simulink model "simulink_model"  (R2023b)
settings: Solver=VariableStepAuto  StartTime=0.0  StopTime=Inf  RelTol=1e-3
values from neighbouring files (symbols this model uses):
  A = [-1.064 1.000; 290.26 0.00]    [model.m]
  B = [-0.25; -331.40]    [model.m]
  C = [-123.34 0.00; 0.00 1.00]    [model.m]
  D = [-13.51; 0]    [model.m]
  dT1 = 0.75    [model.m]
  dT2 = 0.25    [model.m]
  ELEV_INIT = 10000    [model.m]
  ELEV_TARGET = 795    [model.m]
  LAT_INIT = 34.2329    [model.m]
  LAT_OBS = 34.61916    [model.m]
  LAT_TARGET = 34.6588    [model.m]
  LON_INIT = -119.4573    [model.m]
  LON_OBS = -118.8429    [model.m]
  LON_TARGET = -118.769745    [model.m]
  Vel = 1021.08    [model.m]
undefined symbols (not defined in the file or in its folder): Earth, K, L, WGS84
libraries: simulink x3, aerolibtransform2 x1, slpidlib x1, aerolibanimutils x1
settings Model: Creator=Arseni  LastModifiedBy=Arseni

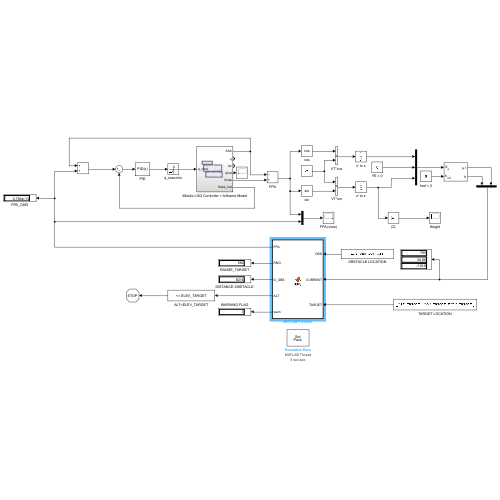
[thumbnail: Simulink's stored preview of the top-level diagram]
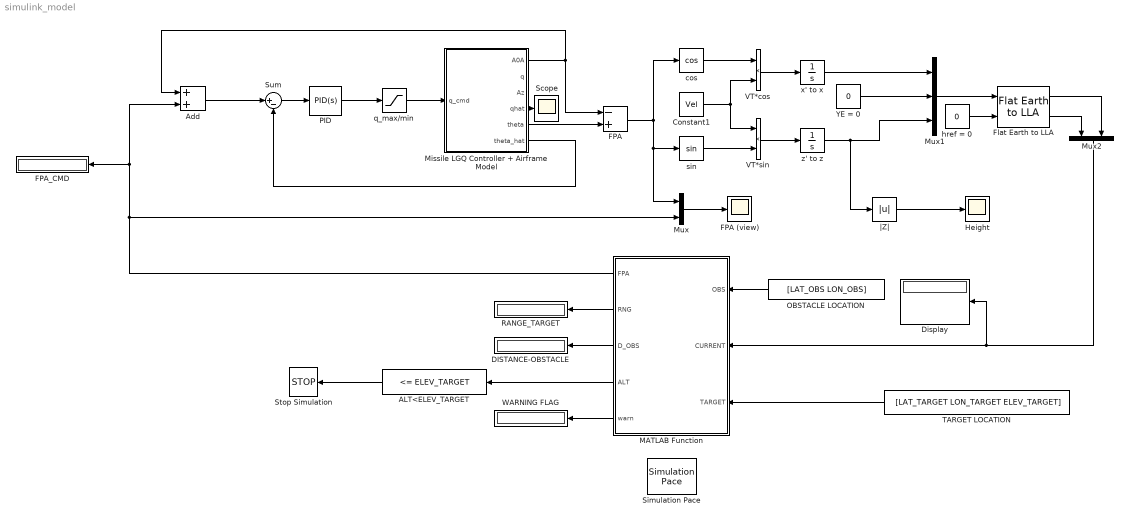
== system simulink_model ==
  ALT<ELEV_TARGET : simulink/Logic and Bit Operations/Compare To Constant  relop=<=  const=ELEV_TARGET  OutDataTypeStr=boolean
  Add : Sum
  Constant1 : Constant  Value=Vel
  DISTANCE-OBSTACLE : Display
  Display : Display
  FPA : Sum  Inputs=-+
  FPA (view) : Scope
  FPA_CMD : Display
  Flat Earth to LLA : aerolibtransform2/Flat Earth to LLA  units=Metric (MKS)  ptype=Earth (WGS84)  F=1/298.257223563  R=6378137  refPosPort=off  LL0=[LAT_INIT LON_INIT]  psi=yaw_init
  Height : Scope
  MATLAB Function : MATLAB Function  TreatAsAtomicUnit=on
  Missile LGQ Controller + Airframe Model : Subsystem
  Mux : Mux  Inputs=2
  Mux1 : Mux  Inputs=3
  Mux2 : Mux  Inputs=2
  OBSTACLE LOCATION : Constant  Value=[LAT_OBS LON_OBS]
  PID : slpidlib/PID Controller  Controller=PID  Form=Parallel  TimeDomain=Continuous-time  UseExternalTs=off  SampleTime=-1  IntegratorMethod=Forward Euler  FilterMethod=Forward Euler  ControllerParametersSource=internal  P=-1  I=0  UseKiTs=off  D=0  N=100  UseFilter=on  TunerSelectOption=Transfer Function Based (PID Tuner App)  InitialConditionSource=internal  InitialConditionForIntegrator=0  InitialConditionForFilter=0  DifferentiatorICPrevScaledInput=0  ExternalReset=none  TrackingMode=off  Kt=1  LimitOutput=off  SatLimitsSource=internal  UpperSaturationLimit=inf  LowerSaturationLimit=-inf  LinearizeAsGain=on  AntiWindupMode=none  Kb=1  LimitIntegrator=off  UpperIntegratorSaturationLimit=inf  LowerIntegratorSaturationLimit=-inf  POutMin=[]  POutMax=[]  IOutMin=[]  IOutMax=[]  DOutMin=[]  DOutMax=[]  NOutMin=[]  NOutMax=[]  SumOutMin=[]  SumOutMax=[]  SaturationOutMin=[]  SaturationOutMax=[]  PParamMin=[]  PParamMax=[]  IParamMin=[]  IParamMax=[]  DParamMin=[]  DParamMax=[]  NParamMin=[]  NParamMax=[]  KbParamMin=[]  KbParamMax=[]  KtParamMin=[]  KtParamMax=[]  KbOutMin=[]  KbOutMax=[]  KtOutMin=[]  KtOutMax=[]  IntegratorOutMin=[]  IntegratorOutMax=[]  FilterOutMin=[]  FilterOutMax=[]  SumI1OutMin=[]  SumI1OutMax=[]  SumI2OutMin=[]  SumI2OutMax=[]  SumI3OutMin=[]  SumI3OutMax=[]  SumI4OutMin=[]  SumI4OutMax=[]  SumDOutMin=[]  SumDOutMax=[]  DifferentiatorOutMin=[]  DifferentiatorOutMax=[]  FilterDiffOutCoefMin=[]  FilterDiffOutCoefMax=[]  ReciprocalOutMin=[]  ReciprocalOutMax=[]  SumDenOutMin=[]  SumDenOutMax=[]  SumNumOutMin=[]  SumNumOutMax=[]  DivideOutMin=[]  DivideOutMax=[]  UdiffTsProdOutMin=[]  UdiffTsProdOutMax=[]  NTsProdOutMin=[]  NTsProdOutMax=[]  UintegralTsProdOutMin=[]  UintegralTsProdOutMax=[]  UngainTsProdOutMin=[]  UngainTsProdOutMax=[]  ClampingZeroOutDataTypeStr=Inherit: Inherit via back propagation  ClampingZeroOutMin=[]  ClampingZeroOutMax=[]  FilterDenConstantOutDataTypeStr=Inherit: Inherit via back propagation  FilterDenConstantOutMin=[]  FilterDenConstantOutMax=[]  PCopyOutDataTypeStr=Inherit: Inherit via back propagation  PCopyOutMin=[]  PCopyOutMax=[]  NCopyOutDataTypeStr=Inherit: Inherit via back propagation  NCopyOutMin=[]  NCopyOutMax=[]  IntegratorContinuousStateAttributes=''  IntegratorStateMustResolveToSignalObject=off  IntegratorRTWStateStorageClass=Auto  FilterContinuousStateAttributes=''  FilterStateMustResolveToSignalObject=off  FilterRTWStateStorageClass=Auto  ParallelPVariant=InternalParameters  IdealPVariant=Disabled  IVariant=InternalParameters  DVariant=InternalParameters  IntegratorVariant=Continuous  SatVariant=Disabled  AWVariant=Passthrough  PCopyVariant=Disabled  TRVariant=Disabled  FdbkBlocksVariant=Forward  IdealPFdbkVariant=Disabled  SatFdbkVariant=Disabled  DerivativeFilterVariant=ContFilter  NVariant=InternalParameters  NCopyVariant=Disabled  FilterICVariant=InternalICsFilter  IntegratorICVariant=InternalICs  ExternalResetVariant=Disabled  TRSumVariant=Passthrough  SumFdbkVariant=Disabled  SumVariant=Sum_PID  TsampFilterVariant=InternalTs  TsampNgainVariant=Passthrough  TsampIntegralVariant=Passthrough  ExternalSaturationOutDataTypeStr=Inherit: Same as second input
  RANGE_TARGET : Display
  Scope : Scope
  Simulation Pace : aerolibanimutils/Simulation Pace  SimulationPace=5  SleepMode=MATLAB Thread  OutputPaceError=off  SampleTime=1/30
  Stop Simulation : Stop
  Sum : Sum  Inputs=|+-
  TARGET LOCATION : Constant  Value=[LAT_TARGET LON_TARGET ELEV_TARGET]
  VT*cos : Product
  VT*sin : Product
  WARNING FLAG : Display
  YE = 0 : Constant  Value=0
  cos : Trigonometry  Operator=cos
  href = 0 : Constant  Value=0
  q_max/min : Saturate
  sin : Trigonometry
  x' to x : Integrator
  z' to z : Integrator  InitialCondition=-ELEV_INIT
  |Z| : Abs  SaturateOnIntegerOverflow=off
  wires:
  PID/1 -> q_max/min/1
  q_max/min/1 -> Missile LGQ Controller + Airframe Model/1(q_cmd)
  Sum/1 -> PID/1
  Missile LGQ Controller + Airframe Model/6(theta_hat) -> Sum/2
  Add/1 -> Sum/1
  Missile LGQ Controller + Airframe Model/5(theta) -> FPA/2
  Missile LGQ Controller + Airframe Model/1(A0A) -> Add/1, FPA/1
  MATLAB Function/1(FPA) -> FPA_CMD/1, Add/2, Mux/2
  FPA/1 -> cos/1, sin/1, Mux/1
  Mux/1 -> FPA (view)/1
  sin/1 -> VT*sin/2
  cos/1 -> VT*cos/1
  Constant1/1 -> VT*sin/1, VT*cos/2
  VT*cos/1 -> x' to x/1
  VT*sin/1 -> z' to z/1
  x' to x/1 -> Mux1/1
  YE = 0/1 -> Mux1/2
  z' to z/1 -> |Z|/1, Mux1/3
  |Z|/1 -> Height/1
  Mux1/1 -> Flat Earth to LLA/1
  href = 0/1 -> Flat Earth to LLA/2
  Flat Earth to LLA/2 -> Mux2/1
  Flat Earth to LLA/1 -> Mux2/2
  OBSTACLE LOCATION/1 -> MATLAB Function/1(OBS)
  Mux2/1 -> MATLAB Function/2(CURRENT), Display/1
  TARGET LOCATION/1 -> MATLAB Function/3(TARGET)
  MATLAB Function/5(warn) -> WARNING FLAG/1
  MATLAB Function/2(RNG) -> RANGE_TARGET/1
  MATLAB Function/3(D_OBS) -> DISTANCE-OBSTACLE/1
  MATLAB Function/4(ALT) -> ALT<ELEV_TARGET/1
  ALT<ELEV_TARGET/1 -> Stop Simulation/1
  Missile LGQ Controller + Airframe Model/4(qhat) -> Scope/1

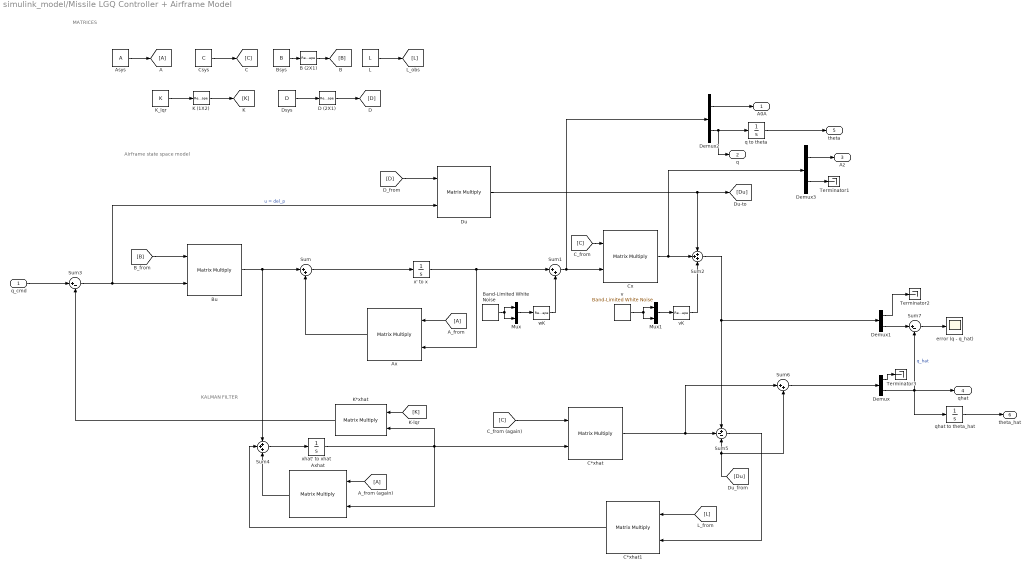
== system simulink_model/Missile LGQ Controller + Airframe Model ==
  note: KALMAN FILTER
  note: Airframe state space model
  note: MATRICES
  q_cmd : Inport
  A : Goto
  A_from : From
  A_from (again) : From
  Asys : Constant  Value=A
  Ax : Product  Multiplication=Matrix(*)
  Axhat : Product  Multiplication=Matrix(*)
  B (2X1) : Reshape  OutputDimensionality=Customize  OutputDimensions=[2,1]
  Band-Limited White Noise : simulink/Sources/Band-Limited White Noise  Cov=0.00000001  Ts=dT1  seed=[23341]
  Bsys : Constant  Value=B
  Bu : Product  Multiplication=Matrix(*)
  C*xhat : Product  Multiplication=Matrix(*)
  C*xhat1 : Product  Multiplication=Matrix(*)
  Csys : Constant  Value=C
  Cx : Product  Multiplication=Matrix(*)
  D (2X1) : Reshape  OutputDimensionality=Customize  OutputDimensions=[2,1]
  Demux{,1..3} (4 alike) : Demux  Outputs=2
  Dsys : Constant  Value=D
  Du : Product  Multiplication=Matrix(*)
  K (1X2) : Reshape  OutputDimensionality=Customize  OutputDimensions=[1,2]
  K*xhat : Product  Multiplication=Matrix(*)
  K_lqr : Constant  Value=K
  L : Constant  Value=L
  Mux : Mux  Inputs=2
  Mux1 : Mux  Inputs=2
  Sum : Sum  Inputs=|++
  Sum1 : Sum  Inputs=|++
  Sum2 : Sum  Inputs=+++
  Sum3 : Sum  Inputs=|+-
  Sum4 : Sum  Inputs=+++
  Sum5 : Sum  Inputs=+--
  Sum6 : Sum  Inputs=|++
  Sum7 : Sum  Inputs=|+-
  Terminator1 : Terminator
  Terminator2 : Terminator
  Terminator3 : Terminator
  error (q - q_hat) : Scope
  q to theta : Integrator
  qhat to theta_hat : Integrator
  v : simulink/Sources/Band-Limited White Noise  Cov=[0.00001]  Ts=dT2  seed=[23341]
  vK : Reshape  OutputDimensionality=Customize  OutputDimensions=[2,1]
  wK : Reshape  OutputDimensionality=Customize  OutputDimensions=[2,1]
  x' to x : Integrator
  xhat' to xhat : Integrator  InitialCondition=[0.01;0.01]
  A0A : Outport
  q : Outport  Port=2
  Az : Outport  Port=3
  qhat : Outport  Port=4
  theta : Outport  Port=5
  theta_hat : Outport  Port=6
  wires:
  C*xhat/1 -> Sum6/1, Sum5/2
  Demux/1 -> Terminator3/1
  B (2X1)/1 -> [B]
  Sum7/1 -> error (q - q_hat)/1
  Ax/1 -> Sum/2
  Sum2/1 -> Demux1/1, Sum5/1
  Du/1 -> Sum2/1, [Du]
  Cx/1 -> Demux3/1, Sum2/2
  Band-Limited White Noise/1 -> Mux/1, Mux/2
  [Du] -> Sum6/2, Sum5/3
  K (1X2)/1 -> [K]
  Demux1/2 -> Sum7/1
  A_from/1 -> Ax/1
  x' to x/1 -> Sum1/1, Ax/2
  q_cmd/1 -> Sum3/1
  [D] -> Du/1
  Sum1/1 -> Cx/2, Demux2/1
  C*xhat1/1 -> Sum4/2
  Sum3/1 -> Bu/2, Du/2  "u = del_p"
  Bu/1 -> Sum/1, Sum4/1
  Demux/2 -> qhat/1, qhat to theta_hat/1, Sum7/2  "q_hat"
  Mux1/1 -> vK/1
  L/1 -> [L]
  Sum/1 -> x' to x/1
  xhat' to xhat/1 -> K*xhat/2, Axhat/2, C*xhat/2
  wK/1 -> Sum1/2
  Csys/1 -> [C]
  Asys/1 -> A/1
  qhat to theta_hat/1 -> theta_hat/1
  v/1 -> Mux1/1, Mux1/2
  D (2X1)/1 -> [D]
  [C] -> C*xhat/1
  Mux/1 -> wK/1
  Demux2/2 -> q/1, q to theta/1
  Demux2/1 -> A0A/1
  Sum4/1 -> xhat' to xhat/1
  [B] -> Bu/1
  Dsys/1 -> D (2X1)/1
  Axhat/1 -> Sum4/3
  q to theta/1 -> theta/1
  Sum6/1 -> Demux/1
  K_lqr/1 -> K (1X2)/1
  Sum5/1 -> C*xhat1/2
  vK/1 -> Sum2/3
  A_from (again)/1 -> Axhat/1
  [C] -> Cx/1
  Demux3/2 -> Terminator1/1
  [K] -> K*xhat/1
  Demux1/1 -> Terminator2/1
  K*xhat/1 -> Sum3/2
  Bsys/1 -> B (2X1)/1
  Demux3/1 -> Az/1
  [L] -> C*xhat1/1

== matlab function simulink_model/MATLAB Function ==
  data: OBS input; FPA output; CURRENT input; TARGET input; RNG output; D_OBS output; ALT output; warn output
function [FPA, RNG, D_OBS, ALT, warn] = fcn(OBS, CURRENT, TARGET)


R = 6371e3;
d2r = pi/180;

% OBSTACLE LOCATION
LAT_OBS = OBS(1);
LON_OBS = OBS(2);

% OBSTACLE THRESHOLD (ZONE)
thres = 2000;

% TARGET LOCATION
LAT_TARGET  = TARGET(1);
LON_TARGET = TARGET(2);
ELEV_TARGET = TARGET(3);

% CURRENT LOCATION
ELEV_CUR = CURRENT(1);
LAT_CUR = CURRENT(2);
LON_CUR = CURRENT(3);

%% distance to target
l1 = LAT_CUR*d2r;
u1 = LON_CUR*d2r;
l2 = LAT_TARGET*d2r;
u2 = LON_TARGET*d2r;
dh = abs(ELEV_TARGET - ELEV_CUR);

dl = l2-l1;
du = u2-u1;

a = sin(dl/2)^2 + cos(l1)*cos(l2)*sin(du/2)^2;
c = 2*atan2(sqrt(a), sqrt(1-a));
d = R*c;  %horizontal distance (in m)

%% distance from the obstacle
l3 = LAT_OBS*d2r;
u3 = LON_OBS*d2r;

dl = l3-l1;
du = u3-u1;

a = sin(dl/2)^2 + cos(l1)*cos(l2)*sin(du/2)^2;
c = 2*atan2(sqrt(a), sqrt(1-a));
d_obs = R*c;  %horizontal distance (in m)

%% current range from the obstacle

range = sqrt(d^2 + dh^2);

%% calculate commanded flight path setpoint based on d_obs, range

if abs(d_obs)>=thres
    w = 0;
    FPA_CMD = atan(dh/d); %rad
else
    %when <2000m, trigger warning
    w = 1;
    FPA_CMD = 0;
end

%% output variables

FPA = FPA_CMD;

RNG = range;

D_OBS = d_obs;

warn = w;

ALT = ELEV_CUR;
